simulink model "odo_trip_demo"  (R2019b)
settings: Solver=ode3  StartTime=0.0  StopTime=1000  FixedStep=0.25  RelTol=1e-3  EnableMultiTasking=on
values from neighbouring files (symbols this model uses):
  km_to_mile = 0.621    [config.m]
  meter_to_km = 1000    [config.m]
  operating_high = 15    [config.m]
  operating_low = 10    [config.m]
  pulse_threshold = 50    [config.m]
  state1_high = 10    [config.m]
  state1_low = 8    [config.m]
  state2_high = 8    [config.m]
  state2_low = 5.9    [config.m]
  state_cpu_reset = 5.9    [config.m]
  wheel_dia_m = 2    [config.m]
undefined symbols (not defined in the file or in its folder): sigbuilder_block, unit_conv
libraries: simulink x1
settings Model: Creator=rajesh.shaw  LastModifiedBy=LCLADMIN
settings DataIOCC: LimitDataPoints=on  SaveFormat=Array  ReturnWorkspaceOutputs=off
settings OptimizationCC: DefaultParameterBehavior=Inlined  EnhancedBackFolding=on  PassReuseOutputArgsAs=Individual arguments  ZeroExternalMemoryAtStartup=off  ZeroInternalMemoryAtStartup=off  OptimizeBlockOrder=speed  DifferentSizesBufferReuse=on  OptimizationCustomize=off  EfficientTunableParamExpr=on
settings DebuggingCC: UnderspecifiedInitializationDetection=Classic  MergeDetectMultiDrivingBlocksExec=none  SolverPrmCheckMsg=warning  ParameterTunabilityLossMsg=error  SFUnexpectedBacktrackingDiag=warning  SFNoUnconditionalDefaultTransitionDiag=warning  SFExecutionAtInitializationDiag=none  ArithmeticOperatorsInVariantConditions=warning
settings HardwareCC: ProdBitPerInt=16  ProdBitPerPointer=16  ProdBitPerSizeT=16  ProdBitPerPtrDiffT=16  ProdLargestAtomicFloat=None  ProdWordSize=16  ProdHWDeviceType=Infineon->C16x, XC16x
settings ModelReferenceCC: PropagateSignalLabelsOutOfModel=off
settings SFSimCC: MATLABDynamicMemAlloc=off  CustomCodeUndefinedFunction=UseInterfaceOnly
settings RTWCC: SystemTargetFile=ert.tlc  TemplateMakefile=ert_default_tmf  GenerateReport=on  IncludeHyperlinkInReport=on  LaunchReport=on  GenerateTraceInfo=on  GenerateTraceReport=on  GenerateTraceReportSl=on  GenerateTraceReportSf=on  GenerateTraceReportEml=on  GenerateWebview=on  GenerateCodeMetricsReport=on
settings CodeAppCC: ForceParamTrailComments=on  IgnoreCustomStorageClasses=off  OperatorAnnotations=on  SimulinkDataObjDesc=on  SFDataObjDesc=on  InsertBlockDesc=on
settings ERTTargetCC: GenerateSampleERTMain=on  InlinedParameterPlacement=NonHierarchical  ERTCustomFileTemplate=example_file_process.tlc
settings ConfigComp: CovEnable=on  RecordCoverage=on  CovMetricSettings=dtrzoibw  CovHtmlReporting=on  CovSaveCumulativeToWorkspaceVar=on  CovSaveSingleToWorkspaceVar=on  CovModelRefEnable=on  CovExternalEMLEnable=off

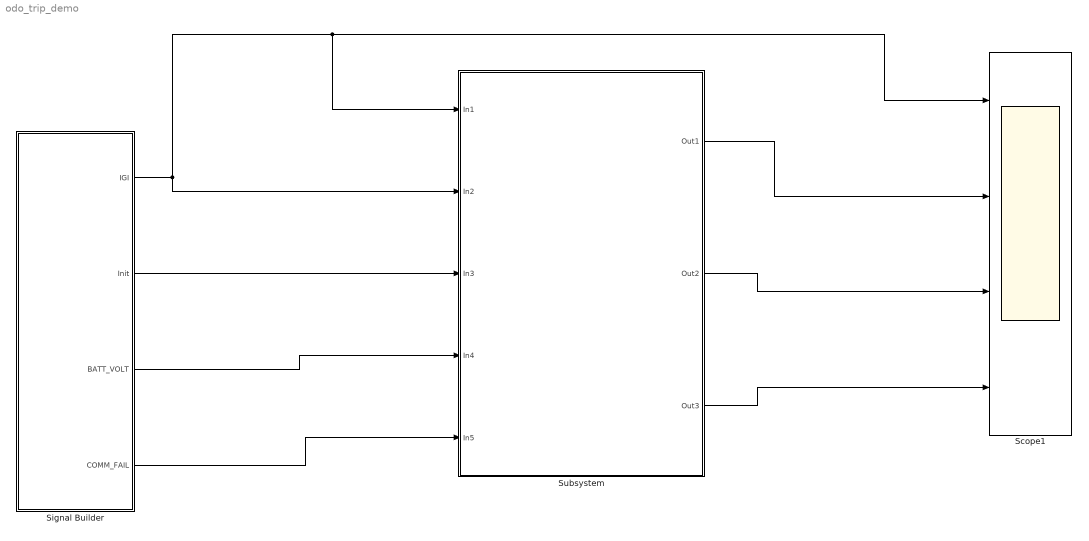
== system odo_trip_demo ==
  Scope1 : Scope  NumInputPorts=4
  Signal Builder : Subsystem  Tag=STV Subsys  LoadFcn=sigbuilder_block('load');  StartFcn=sigbuilder_block('start');  StopFcn=sigbuilder_block('stop');  ClipboardFcn=sigbuilder_block('clipboard');  mask(Sigbuilder block){tuvar=[0:10]}
      mask help: Simulink:masks:SigbuilderBlock_MD
      mask init:
      | if ~strcmp(get_param(bdroot(gcbh),'SimulationStatus'),'stopped') tuvar = sigbuilder_block('maskInit'); end
      settings: CopyFcn=sigbuilder_block('copy');  DeleteFcn=sigbuilder_block('delete');  ModelCloseFcn=sigbuilder_block('modelClose');  PreSaveFcn=sigbuilder_block('preSave');  PauseFcn=sigbuilder_block('pause');  ContinueFcn=sigbuilder_block('continue');  NameChangeFcn=sigbuilder_block('namechange');  OpenFcn=sigbuilder_block('open',[437.25 117.75 550.5 394.5 ]);  CloseFcn=sigbuilder_block('close');
      mask Display: plot(0, 0, 100, 100,[2, 2, 32, 32, 2], [68, 8, 8, 68, 68],[32, 2], [38, 38], [32, 19, 2],[53, 60, 44], [32, 17, 17, 2],[16, 16, 31, 31]);txt = getActiveGroup(gcbh);text(2, 100, txt,'verticalAlignment', 'top');
  Subsystem : Subsystem
  wires:
  Signal Builder/1(IGI) -> Subsystem/1(In1), Scope1/1, Subsystem/2(In2)
  Signal Builder/2(Init) -> Subsystem/3(In3)
  Signal Builder/3(BATT_VOLT) -> Subsystem/4(In4)
  Signal Builder/4(COMM_FAIL) -> Subsystem/5(In5)
  Subsystem/1(Out1) -> Scope1/2
  Subsystem/2(Out2) -> Scope1/3
  Subsystem/3(Out3) -> Scope1/4

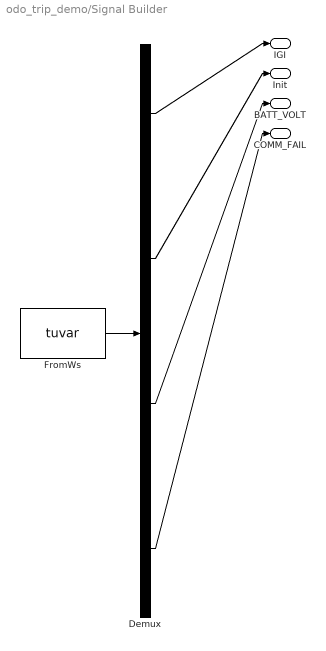
== system odo_trip_demo/Signal Builder ==
  Demux : Demux  Tag=STV Demux
  FromWs : FromWorkspace  Tag=STV FromWs  VariableName=tuvar  SampleTime=0
      SigBuilderData=|
      | common.afterFinalStr = 'Extrapolate'
      | common.sampleTime = 0
      | dataSet.timeRange = [0 1000]
      | dataSet.name = 'Group 1'
      | sbobj.Groups.Name = 'Group 1'
      | sbobj.Groups.Signals(1).Name = 'IGI'
      | sbobj.Groups.Signals(1).XData = [0 10 10 1000]
      | sbobj.Groups.Signals(1).YData = [0 0 1 1]
      | sbobj.Groups.Signals(2).Name = 'Init'
      | sbobj.Groups.Signals(2).XData = [0 10.5 10.5 1000]
      | sbobj.Groups.Signals(2).YData = [1 1 0 0]
      | sbobj.Groups.Signals(3).Name = 'BATT_VOLT'
      | sbobj.Groups.Signals(3).XData = [0 20 20 1000]
      | sbobj.Groups.Signals(3).YData = [0 0 12 12]
      | sbobj.Groups.Signals(4).Name = 'COMM_FAIL'
      | sbobj.Groups.Signals(4).XData = [0 800 800 850 850 1000]
      | sbobj.Groups.Signals(4).YData = [0 0 1 1 0 0]
      | sbobj.Groups.TimeRange = [0 1000]
  IGI : Outport  Tag=STV Outport  VectorParamsAs1DForOutWhenUnconnected=off
  Init : Outport  Tag=STV Outport  Port=2  VectorParamsAs1DForOutWhenUnconnected=off
  BATT_VOLT : Outport  Tag=STV Outport  Port=3  VectorParamsAs1DForOutWhenUnconnected=off
  COMM_FAIL : Outport  Tag=STV Outport  Port=4  VectorParamsAs1DForOutWhenUnconnected=off
  wires:
  FromWs/1 -> Demux/1
  Demux/1 -> IGI/1
  Demux/2 -> Init/1
  Demux/3 -> BATT_VOLT/1
  Demux/4 -> COMM_FAIL/1

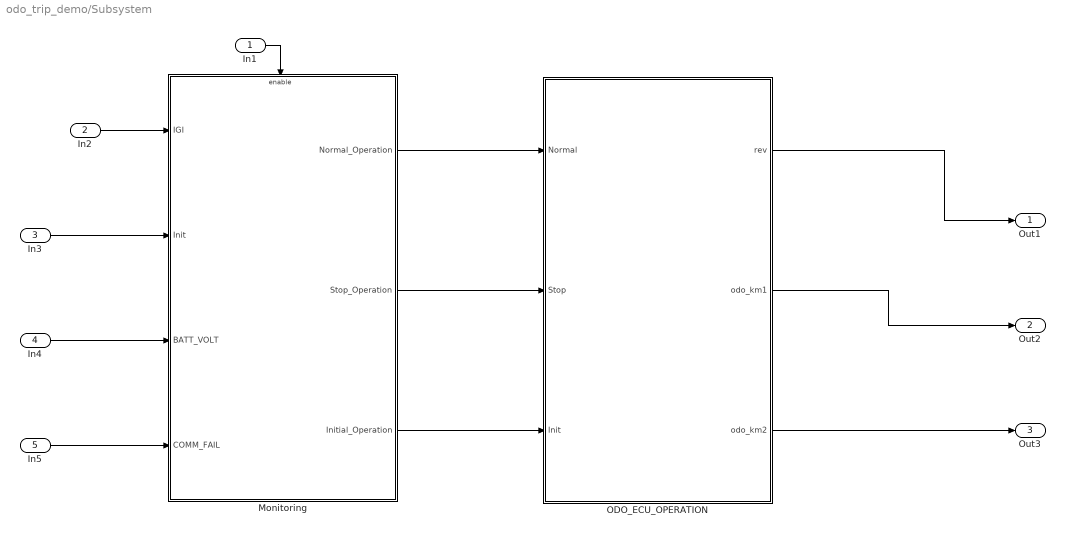
== system odo_trip_demo/Subsystem ==
  In1 : Inport
  In2 : Inport  Port=2
  In3 : Inport  Port=3  PortDimensions=4
  In4 : Inport  Port=4
  In5 : Inport  Port=5
  Monitoring : Subsystem  TreatAsAtomicUnit=on
  ODO_ECU_OPERATION : Subsystem
  Out1 : Outport
  Out2 : Outport  Port=2
  Out3 : Outport  Port=3
  wires:
  ODO_ECU_OPERATION/1(rev) -> Out1/1
  ODO_ECU_OPERATION/3(odo_km2) -> Out3/1
  Monitoring/1(Normal_Operation) -> ODO_ECU_OPERATION/1(Normal)
  Monitoring/3(Initial_Operation) -> ODO_ECU_OPERATION/3(Init)
  In1/1 -> Monitoring/Enable
  In5/1 -> Monitoring/4(COMM_FAIL)
  In4/1 -> Monitoring/3(BATT_VOLT)
  ODO_ECU_OPERATION/2(odo_km1) -> Out2/1
  Monitoring/2(Stop_Operation) -> ODO_ECU_OPERATION/2(Stop)
  In3/1 -> Monitoring/2(Init)
  In2/1 -> Monitoring/1(IGI)

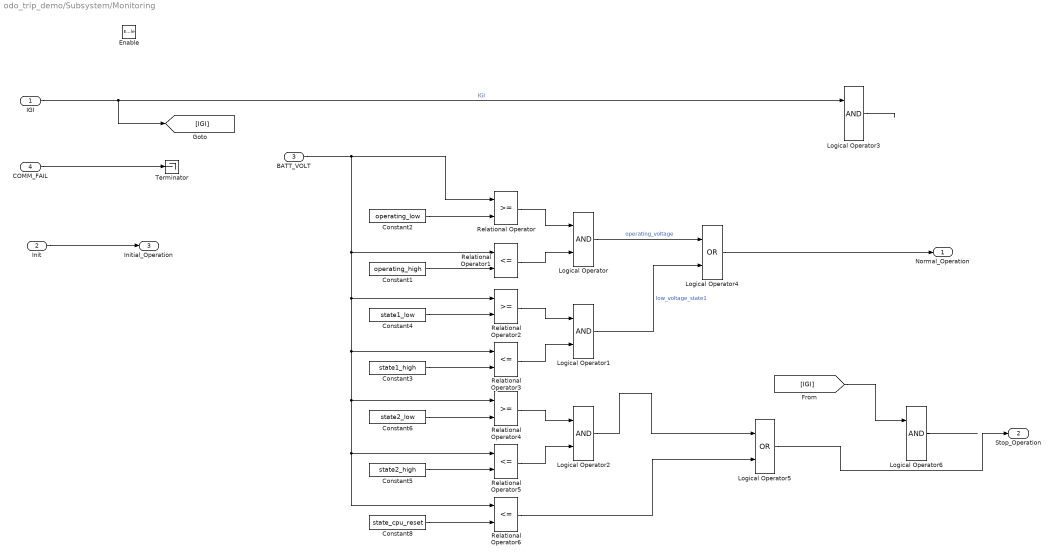
== system odo_trip_demo/Subsystem/Monitoring ==
  IGI : Inport
  Init : Inport  Port=2
  BATT_VOLT : Inport  Port=3
  COMM_FAIL : Inport  Port=4
  Enable : EnablePort
  Constant1 : Constant  Value=operating_high
  Constant2 : Constant  Value=operating_low
  Constant3 : Constant  Value=state1_high
  Constant4 : Constant  Value=state1_low
  Constant5 : Constant  Value=state2_high
  Constant6 : Constant  Value=state2_low
  Constant8 : Constant  Value=state_cpu_reset
  Logical Operator{,1..3,6} (5 alike) : Logic  AllPortsSameDT=off  OutDataTypeStr=boolean
  Logical Operator4 : Logic  Operator=OR  AllPortsSameDT=off  OutDataTypeStr=boolean
  Logical Operator5 : Logic  Operator=OR  AllPortsSameDT=off  OutDataTypeStr=boolean
  Relational Operator : RelationalOperator  OutDataTypeStr=boolean  RndMeth=Nearest
  Relational Operator{1,3,5..6} (4 alike) : RelationalOperator  Operator=<=  OutDataTypeStr=boolean  RndMeth=Nearest
  Relational Operator2 : RelationalOperator  OutDataTypeStr=boolean  RndMeth=Nearest
  Relational Operator4 : RelationalOperator  OutDataTypeStr=boolean  RndMeth=Nearest
  Terminator : Terminator
  Normal_Operation : Outport  VectorParamsAs1DForOutWhenUnconnected=off
  Stop_Operation : Outport  Port=2  VectorParamsAs1DForOutWhenUnconnected=off
  Initial_Operation : Outport  Port=3  VectorParamsAs1DForOutWhenUnconnected=off
  wires:
  Constant2/1 -> Relational Operator/2
  Constant1/1 -> Relational Operator1/2
  Constant4/1 -> Relational Operator2/2
  Constant3/1 -> Relational Operator3/2
  Constant6/1 -> Relational Operator4/2
  Constant5/1 -> Relational Operator5/2
  BATT_VOLT/1 -> Relational Operator1/1, Relational Operator2/1, Relational Operator6/1, Relational Operator5/1, Relational Operator4/1, Relational Operator3/1, Relational Operator/1
  Constant8/1 -> Relational Operator6/2
  Relational Operator1/1 -> Logical Operator/2
  Relational Operator/1 -> Logical Operator/1
  Relational Operator2/1 -> Logical Operator1/1
  Relational Operator3/1 -> Logical Operator1/2
  Relational Operator4/1 -> Logical Operator2/1
  Relational Operator5/1 -> Logical Operator2/2
  Relational Operator6/1 -> Logical Operator5/2
  Logical Operator2/1 -> Logical Operator5/1
  Logical Operator1/1 -> Logical Operator4/2  "low_voltage_state1"
  IGI/1 -> [IGI], Logical Operator3/1  "IGI"
  Logical Operator/1 -> Logical Operator4/1  "operating_voltage"
  Logical Operator4/1 -> Normal_Operation/1
  [IGI] -> Logical Operator6/1
  Logical Operator5/1 -> Stop_Operation/1
  COMM_FAIL/1 -> Terminator/1
  Logical Operator3/1 -> ?
  Logical Operator6/1 -> ?
  Init/1 -> Initial_Operation/1

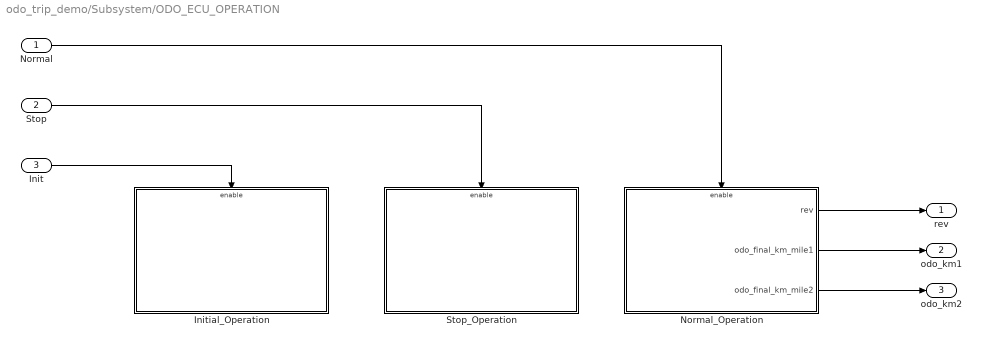
== system odo_trip_demo/Subsystem/ODO_ECU_OPERATION ==
  Normal : Inport
  Stop : Inport  Port=2
  Init : Inport  Port=3
  Initial_Operation : Subsystem
  Normal_Operation : Subsystem
  Stop_Operation : Subsystem
  rev : Outport  VectorParamsAs1DForOutWhenUnconnected=off
  odo_km1 : Outport  Port=2  VectorParamsAs1DForOutWhenUnconnected=off
  odo_km2 : Outport  Port=3  VectorParamsAs1DForOutWhenUnconnected=off
  wires:
  Normal_Operation/2(odo_final_km_mile1) -> odo_km1/1
  Init/1 -> Initial_Operation/Enable
  Normal_Operation/1(rev) -> rev/1
  Normal/1 -> Normal_Operation/Enable
  Stop/1 -> Stop_Operation/Enable
  Normal_Operation/3(odo_final_km_mile2) -> odo_km2/1

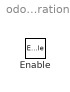
== system odo_trip_demo/Subsystem/ODO_ECU_OPERATION/Initial_Operation ==
  Enable : EnablePort

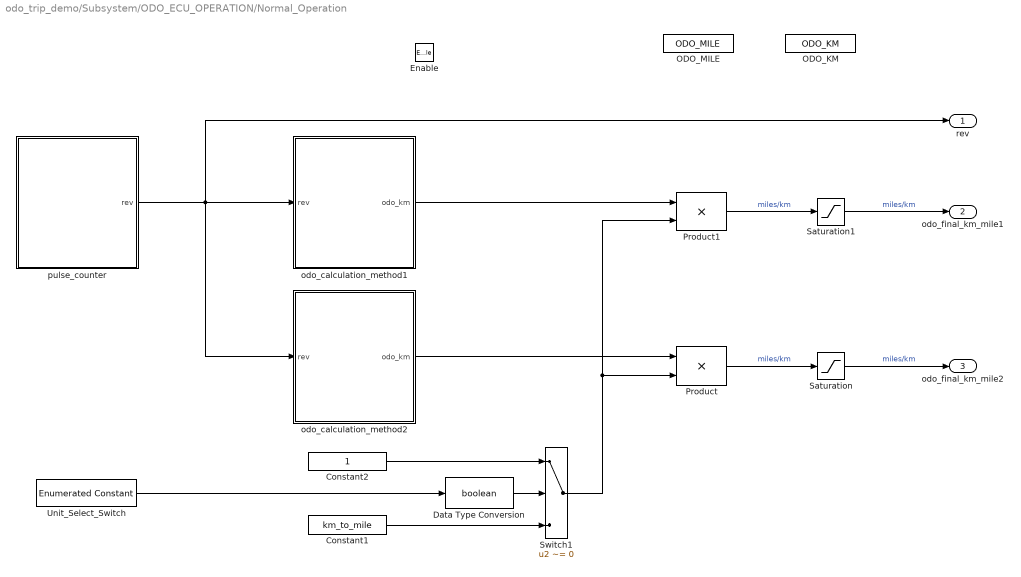
== system odo_trip_demo/Subsystem/ODO_ECU_OPERATION/Normal_Operation ==
  Enable : EnablePort
  Constant1 : Constant  Value=km_to_mile
  Constant2 : Constant
  Data Type Conversion : DataTypeConversion  OutDataTypeStr=boolean
  ODO_KM : DataStoreMemory  DataStoreName=ODO_KM  ReadBeforeWriteMsg=warning  WriteAfterWriteMsg=warning  WriteAfterReadMsg=warning  ShowAdditionalParam=off
  ODO_MILE : DataStoreMemory  DataStoreName=ODO_MILE  ReadBeforeWriteMsg=warning  WriteAfterWriteMsg=warning  WriteAfterReadMsg=warning  ShowAdditionalParam=off
  Product : Product
  Product1 : Product
  Saturation : Saturate  UpperLimit=999999  LowerLimit=0
  Saturation1 : Saturate  UpperLimit=999999  LowerLimit=0
  Switch1 : Switch  Criteria=u2 ~= 0
  Unit_Select_Switch : simulink/Sources/Enumerated Constant  OutDataTypeStr=Enum: unit_conv  Value=unit_conv.Unit_KM  SampleTime=inf
      settings: SourceProductName=Simulink
  odo_calculation_method1 : Subsystem
  odo_calculation_method2 : Subsystem
  pulse_counter : Subsystem  TreatAsAtomicUnit=on
  rev : Outport  VectorParamsAs1DForOutWhenUnconnected=off
  odo_final_km_mile1 : Outport  Port=2  VectorParamsAs1DForOutWhenUnconnected=off
  odo_final_km_mile2 : Outport  Port=3  VectorParamsAs1DForOutWhenUnconnected=off
  wires:
  Constant2/1 -> Switch1/1
  odo_calculation_method1/1(odo_km) -> Product1/1
  Switch1/1 -> Product1/2, Product/2
  Product/1 -> Saturation/1  "miles/km"
  Constant1/1 -> Switch1/3
  Unit_Select_Switch/1 -> Data Type Conversion/1
  pulse_counter/1(rev) -> odo_calculation_method2/1(rev), odo_calculation_method1/1(rev), rev/1
  odo_calculation_method2/1(odo_km) -> Product/1
  Data Type Conversion/1 -> Switch1/2
  Saturation/1 -> odo_final_km_mile2/1  "miles/km"
  Saturation1/1 -> odo_final_km_mile1/1  "miles/km"
  Product1/1 -> Saturation1/1  "miles/km"

== system odo_trip_demo/Subsystem/ODO_ECU_OPERATION/Stop_Operation ==
  Enable : EnablePort

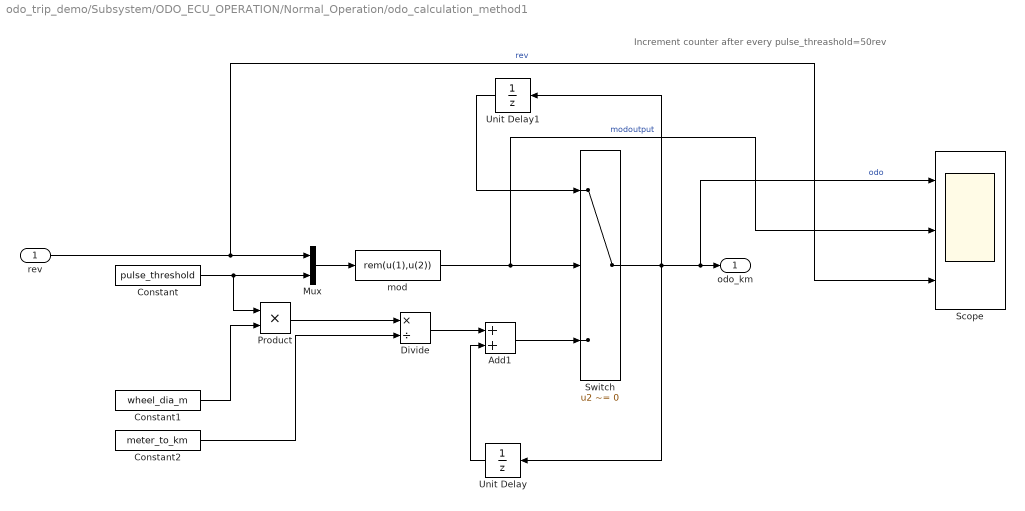
== system odo_trip_demo/Subsystem/ODO_ECU_OPERATION/Normal_Operation/odo_calculation_method1 ==
  note: Increment counter after every pulse_threashold=50rev
  rev : Inport
  Add1 : Sum
  Constant : Constant  Value=pulse_threshold
  Constant1 : Constant  Value=wheel_dia_m
  Constant2 : Constant  Value=meter_to_km
  Divide : Product  Inputs=*/
  Mux : Mux  Inputs=2
  Product : Product
  Scope : Scope  NumInputPorts=3
  Switch : Switch  Criteria=u2 ~= 0
  Unit Delay : UnitDelay  SampleTime=-1  HasFrameUpgradeWarning=on
  Unit Delay1 : UnitDelay  SampleTime=-1  HasFrameUpgradeWarning=on
  mod : Fcn  Expr=rem(u(1),u(2))
  odo_km : Outport  VectorParamsAs1DForOutWhenUnconnected=off
  wires:
  Constant/1 -> Product/1, Mux/2
  mod/1 -> Scope/2, Switch/2  "modoutput"
  rev/1 -> Scope/3, Mux/1  "rev"
  Switch/1 -> Unit Delay/1, Unit Delay1/1, Scope/1, odo_km/1  "odo"
  Mux/1 -> mod/1
  Unit Delay1/1 -> Switch/1
  Constant1/1 -> Product/2
  Product/1 -> Divide/1
  Constant2/1 -> Divide/2
  Divide/1 -> Add1/1
  Unit Delay/1 -> Add1/2
  Add1/1 -> Switch/3

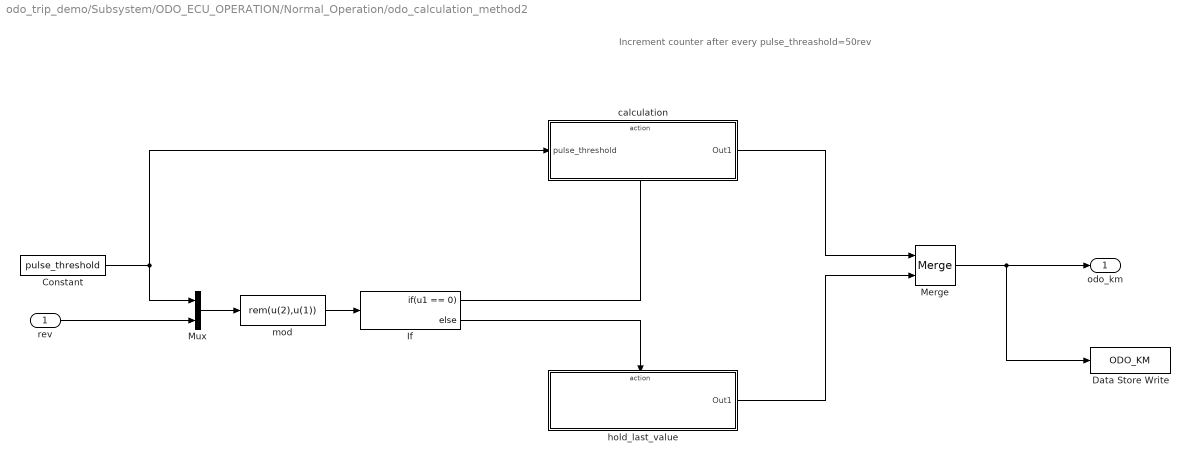
== system odo_trip_demo/Subsystem/ODO_ECU_OPERATION/Normal_Operation/odo_calculation_method2 ==
  note: Increment counter after every pulse_threashold=50rev
  rev : Inport
  Constant : Constant  Value=pulse_threshold
  Data Store Write : DataStoreWrite  DataStoreName=ODO_KM
  If : If  IfExpression=u1 == 0
  Merge : Merge
  Mux : Mux  Inputs=2
  calculation : Subsystem  TreatAsAtomicUnit=on
  hold_last_value : Subsystem  TreatAsAtomicUnit=on
  mod : Fcn  Expr=rem(u(2),u(1))
  odo_km : Outport  VectorParamsAs1DForOutWhenUnconnected=off
  wires:
  Mux/1 -> mod/1
  If/1 -> calculation/Action
  Constant/1 -> calculation/1(pulse_threshold), Mux/1
  mod/1 -> If/1
  If/2 -> hold_last_value/Action
  Merge/1 -> Data Store Write/1, odo_km/1
  calculation/1(Out1) -> Merge/1
  hold_last_value/1(Out1) -> Merge/2
  rev/1 -> Mux/2

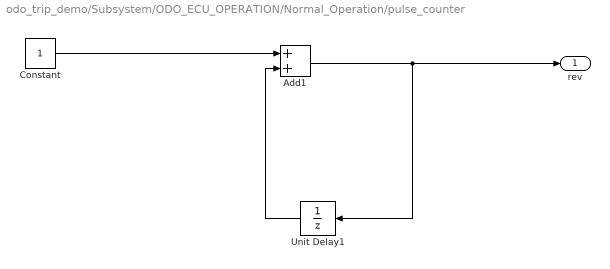
== system odo_trip_demo/Subsystem/ODO_ECU_OPERATION/Normal_Operation/pulse_counter ==
  Add1 : Sum
  Constant : Constant
  Unit Delay1 : UnitDelay  SampleTime=-1  HasFrameUpgradeWarning=on
  rev : Outport  VectorParamsAs1DForOutWhenUnconnected=off
  wires:
  Add1/1 -> rev/1, Unit Delay1/1
  Unit Delay1/1 -> Add1/2
  Constant/1 -> Add1/1

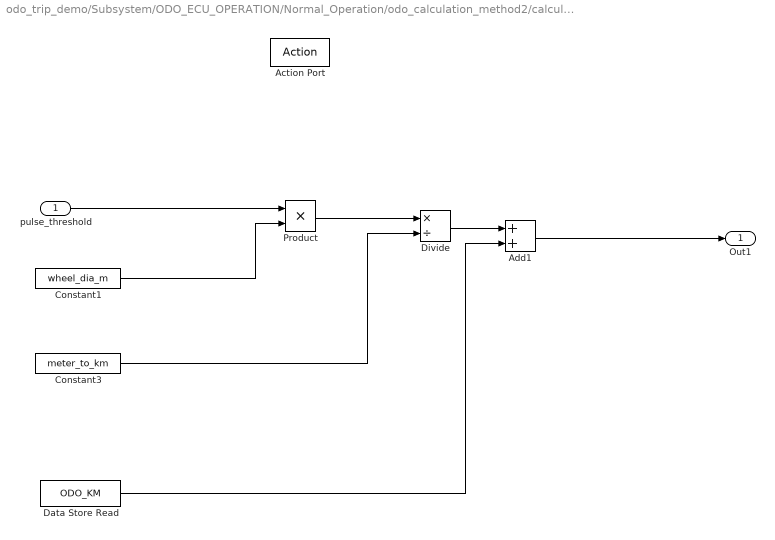
== system odo_trip_demo/Subsystem/ODO_ECU_OPERATION/Normal_Operation/odo_calculation_method2/calculation ==
  pulse_threshold : Inport
  Action Port : ActionPort  ActionPortLabel=if(u1 == 0)
  Add1 : Sum
  Constant1 : Constant  Value=wheel_dia_m
  Constant3 : Constant  Value=meter_to_km
  Data Store Read : DataStoreRead  DataStoreName=ODO_KM
  Divide : Product  Inputs=*/
  Product : Product
  Out1 : Outport  VectorParamsAs1DForOutWhenUnconnected=off
  wires:
  Add1/1 -> Out1/1
  Divide/1 -> Add1/1
  Product/1 -> Divide/1
  Constant1/1 -> Product/2
  pulse_threshold/1 -> Product/1
  Data Store Read/1 -> Add1/2
  Constant3/1 -> Divide/2

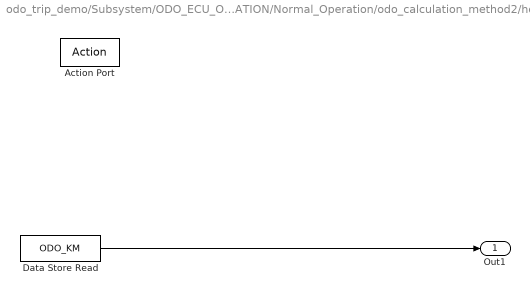
== system odo_trip_demo/Subsystem/ODO_ECU_OPERATION/Normal_Operation/odo_calculation_method2/hold_last_value ==
  Action Port : ActionPort  ActionPortLabel=else
  Data Store Read : DataStoreRead  DataStoreName=ODO_KM
  Out1 : Outport  VectorParamsAs1DForOutWhenUnconnected=off
  wires:
  Data Store Read/1 -> Out1/1
